simulink model "variable_rafael"  (Simulink 8.0)
settings: Solver=ode45  StartTime=0  StopTime=50  FixedStep=0.01  RelTol=0.001
libraries: fmu_me_1_0_lib x1
settings Model: Creator=luigiv  LastModifiedBy=Tin Rabuzin
settings DataIOCC: SignalLoggingSaveFormat=ModelDataLogs  OutputSaveName=simout
settings DebuggingCC: FcnCallInpInsideContextMsg=EnableAllAsWarning
settings GRTTargetCC: CombineOutputUpdateFcns=off  GRTInterface=on

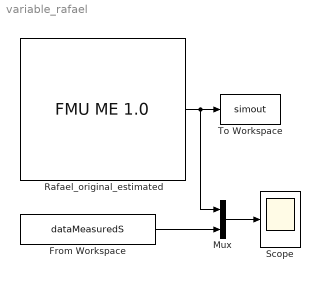
== system variable_rafael ==
  From Workspace : FromWorkspace  VariableName=dataMeasuredS
  Mux : Mux  Inputs=2
  Rafael_original_estimated : fmu_me_1_0_lib/FMU ME 1.0  Description=Simulates an FMU for model exchange 1.0.
  Scope : Scope
      settings: TimeRange=50  YMin=0  YMax=0.4
  To Workspace : ToWorkspace  VariableName=simout  SampleTime=-1  SaveFormat=Structure With Time
  wires:
  Rafael_original_estimated/1 -> To Workspace/1, Mux/1
  Mux/1 -> Scope/1
  From Workspace/1 -> Mux/2
